simulink model "EJ_01_v18_02"  (R2018a)
settings: Solver=ode23t  StartTime=0.0  StopTime=5  FixedStep=0.01  MaxStep=0.05  RelTol=1e-3  EnableMultiTasking=on
PreLoadFcn:
  | mdl_puma560
values from neighbouring files (symbols this model uses):
  messi = SerialLink([links{:}], 'tool', Tool, 'name', 'messi')    [Ej_01.m]
  q0 = [0 -pi/2]    [Ej_01.m]
undefined symbols (not defined in the file or in its folder): jacob0, my_jacob, slcoulomb, vector_sweep
libraries: roblocks x5, dspmtrx3 x1
settings Model: ExtModeTrigMode=oneshot  ExtModeArmWhenConnect=off  Creator=pic  LastModifiedBy=sebas
settings SolverCC: ZeroCrossControl=DisableAll
settings DataIOCC: SaveFormat=Array  SignalLoggingSaveFormat=ModelDataLogs  ReturnWorkspaceOutputs=on  TimeSaveName=t  OutputSaveName=y  ReturnWorkspaceOutputsName=ctorque
settings OptimizationCC: BlockReduction=off  BooleanDataType=off  ExpressionDepthLimit=2147483647  InitFltsAndDblsToZero=on  LifeSpan=inf
settings DebuggingCC: SaveWithParameterizedLinksMsg=none  UnderspecifiedInitializationDetection=Classic  MergeDetectMultiDrivingBlocksExec=none  SignalResolutionControl=TryResolveAllWithWarning  MultiTaskDSMMsg=warning  MultiTaskCondExecSysMsg=none  FcnCallInpInsideContextMsg=warning  AllowSymbolicDim=off  StateNameClashWarn=warning  SFUnexpectedBacktrackingDiag=warning  SFNoUnconditionalDefaultTransitionDiag=warning  SFExecutionAtInitializationDiag=none
settings HardwareCC: ProdBitPerPointer=32  ProdBitPerSizeT=32  ProdBitPerPtrDiffT=32  ProdLargestAtomicFloat=None  ProdIntDivRoundTo=Undefined  ProdEndianess=Unspecified  ProdWordSize=32  ProdHWDeviceType=32-bit Generic  TargetUnknown=on
settings ModelReferenceCC: PropagateSignalLabelsOutOfModel=off
settings CodeAppCC: StateflowObjectComments=on
settings GRTTargetCC: TargetLangStandard=C89/C90 (ANSI)  ModelReferenceCompliant=off  CompOptLevelCompliant=off  GeneratePreprocessorConditionals=Disable all  CombineOutputUpdateFcns=off  MatFileLogging=off  GRTInterface=on
settings ConfigComp: CovMetricSettings=dw  CovHtmlReporting=on  CovSaveCumulativeToWorkspaceVar=on  CovSaveSingleToWorkspaceVar=on  CovExternalEMLEnable=off

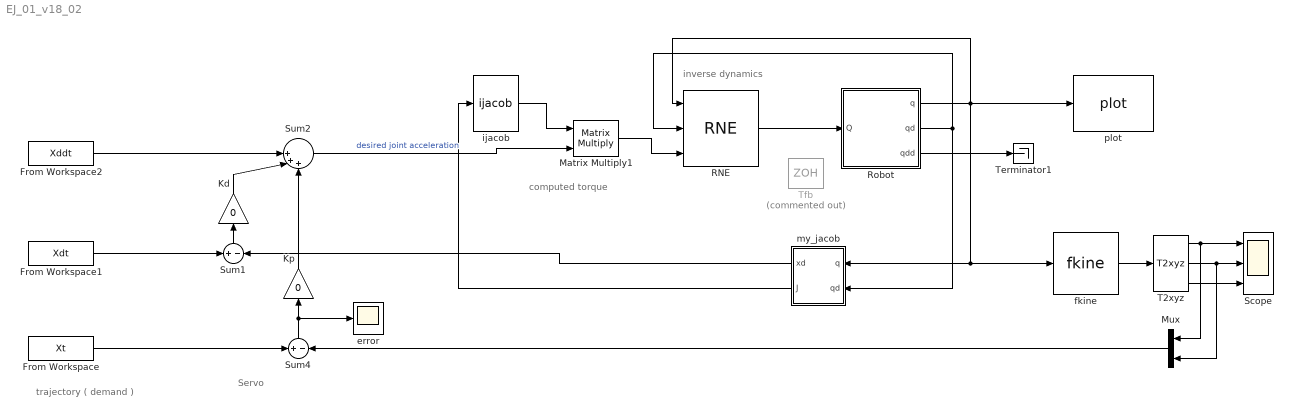
== system EJ_01_v18_02 ==
  note: inverse dynamics
  note: computed torque
  note: trajectory
      | ( demand )
  note: Servo
  From Workspace : FromWorkspace  VariableName=Xt
  From Workspace1 : FromWorkspace  VariableName=Xdt
  From Workspace2 : FromWorkspace  VariableName=Xddt
  Kd : Gain  Gain=0  SaturateOnIntegerOverflow=on  OutDataTypeStr=Inherit: Same as input  ParamDataTypeStr=Inherit: Same as input
  Kp : Gain  Gain=0  SaturateOnIntegerOverflow=on  OutDataTypeStr=Inherit: Same as input  ParamDataTypeStr=Inherit: Same as input
  Matrix Multiply1 : Product  Multiplication=Matrix(*)
  Mux : Mux  Inputs=2
  RNE : roblocks/Arm/RNE  robot=messi  grav=[0 0 9.81]
  Robot : Subsystem  AncestorBlock=roblocks/Arm/Robot  mask{robot=messi, q0=q0}
      mask prompts: robot "Robot object"; q0 "Initial state"
      mask help: Rigid-body dynamic model of robot.
      mask init:
      | if isa(robot, 'SerialLink')
      |     rname = robot.name;
      |     %fprintf('**robot name is %s\n', rname);
      | else
      |     rname = '';
      |     n = 0
      | end
      mask Help:
      | Simulates the forward (direct) rigid-body dynamics of the robot described
      | by the given robot object.  For given applied joint torque/force it computes
      | the instaneous joint coordinates, velocities and acclerations.
      | 
      | 
      | <b>Parameters::</b>
      | 
      | robot (SerialLink) a dynamic model of an N-link serial link manipulator
      | q0 (1xN)  Initial joint coordinates
      | 
      | <b>Inputs::</b>
      | 
      | Q (1xN) the generalized joint force (torque or force) required to achieve
      | the motion state (q, qd, qdd).
      | 
      | <b>Outputs::</b>
      | 
      | q (1xN) joint coordinates
      | qd (1xN) joint coordinate velocity
      | qdd (1xN) joint coordinate acceleration
      | 
      | 
      | <b>Notes::</b>
      | 
      | - Required to simulate robot rigid body motion.
      | - Implemented using the recursive Newton-Euler scheme (RNE).
      | - A wrapper for the Toolbox method accel() which in turn depends on the
      |   method rne().
      mask Display:
      | port_label('input', 1, 'Q')
      | port_label('output', 1, 'q')
      | port_label('output', 2, 'qd')
      | port_label('output', 3, 'qdd')
      | text(0.1, 0.9,  rname, 'horizontalAlignment', 'left')
  Scope : Scope  NumInputPorts=3
  Sum1 : Sum  Inputs=+|-  SaturateOnIntegerOverflow=on  InputSameDT=on  OutDataTypeStr=Inherit: Same as first input
  Sum2 : Sum  Inputs=||+++  SaturateOnIntegerOverflow=on  InputSameDT=on  OutDataTypeStr=Inherit: Same as first input
  Sum4 : Sum  Inputs=+|-  SaturateOnIntegerOverflow=on  InputSameDT=on  OutDataTypeStr=Inherit: Same as first input
  T2xyz : roblocks/Toolbox/T2xyz
  Terminator1 : Terminator
  Tfb : ZeroOrderHold  Commented=on  SampleTime=0.005
  error : Scope
  fkine : roblocks/Arm/fkine  robot=messi
  ijacob : roblocks/Arm/ijacob
  "my_jacob " : Subsystem  AncestorBlock=vector_sweep/my_jacob  mask{robot=messi}
      mask prompts: robot "Robot object"
      mask help: Robot Jacobian in world coordinates
      mask init:
      | n=robot.n;
      mask Help:
      | Jacobian matrix relating joint coordinate rates to end-effector spatial
      | velocity expressed in the world frame.
      | 
      | <b>Parameters::</b>
      | 
      | Robot (SerialLink class)  The N-axis robot object for which the Jacobian is
      |                           computed.
      | 
      | <b>Inputs::</b>
      | 
      | q (1xN) joint coordinates
      | 
      | <b>Outputs::</b>
      | 
      | J (6xN) the Jacobian matrix
      | 
      | <b>Notes::</b>
      | 
      | - A wrapper for the Toolbox method jacob0().
      mask Display:
      | text(0.4, 0.7, '\bf\fontsize{16}J', 'texmode', 'on', 'verticalAlignment', 'top', 'horizontalAlignment', 'left')
      | text(0.45, 0.65, '\fontsize{10}0', 'texmode', 'on','verticalAlignment', 'bottom', 'horizontalAlignment', 'right')
      | if ~isempty(robot)
      |     text(0.5, 0.2, robot.name,  'horizontalAlignment', 'center')
      | end
      | port_label('input', 1, 'q')
      | port_label('input', 2, 'qd')
      | port_label('output', 1, 'xd')
  plot : roblocks/Arm/plot  robot=messi  fps=10  holdplot=on
  wires:
  Robot/3(qdd) -> Terminator1/1
  fkine/1 -> T2xyz/1
  T2xyz/3 -> Scope/3
  T2xyz/2 -> Mux/2, Scope/2
  T2xyz/1 -> Mux/1, Scope/1
  Sum1/1 -> Kd/1
  Sum4/1 -> Kp/1, error/1
  From Workspace/1 -> Sum4/1
  From Workspace1/1 -> Sum1/1
  Kp/1 -> Sum2/3
  Kd/1 -> Sum2/2
  From Workspace2/1 -> Sum2/1
  RNE/1 -> Robot/1(Q)
  Mux/1 -> Sum4/2
  "my_jacob "/1(xd) -> Sum1/2
  ijacob/1 -> Matrix Multiply1/1
  Sum2/1 -> Matrix Multiply1/2  "desired joint acceleration"
  Matrix Multiply1/1 -> RNE/3
  Robot/1(q) -> plot/1, fkine/1, "my_jacob "/1(q), RNE/1
  Robot/2(qd) -> "my_jacob "/2(qd), RNE/2
  "my_jacob "/2(J) -> ijacob/1

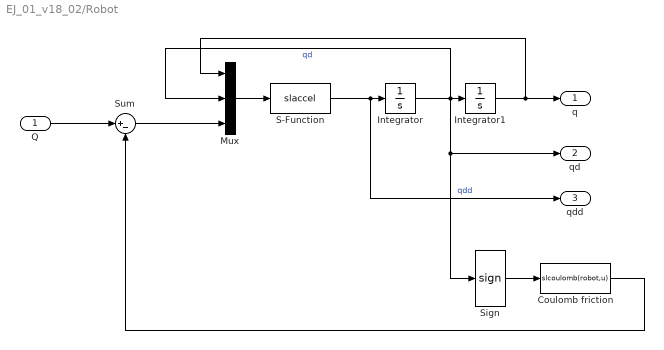
== system EJ_01_v18_02/Robot ==
  Q : Inport
  Coulomb friction : MATLABFcn  MATLABFcn=slcoulomb(robot,u)  OutputDimensions=[robot.n 1]  Output1D=off
  Integrator : Integrator
  Integrator1 : Integrator  InitialCondition=q0
  Mux : Mux  Inputs=3
  S-Function : S-Function  FunctionName=slaccel  Parameters=robot  SFunctionDeploymentMode=off  EnableBusSupport=off
  Sign : Signum
  Sum : Sum  Inputs=|+-
  q : Outport
  qd : Outport  Port=2
  qdd : Outport  Port=3
  wires:
  S-Function/1 -> qdd/1, Integrator/1  "qdd"
  Mux/1 -> S-Function/1
  Integrator/1 -> Sign/1, qd/1, Integrator1/1, Mux/2  "qd"
  Integrator1/1 -> q/1, Mux/1
  Q/1 -> Sum/1
  Sum/1 -> Mux/3
  Coulomb friction/1 -> Sum/2
  Sign/1 -> Coulomb friction/1

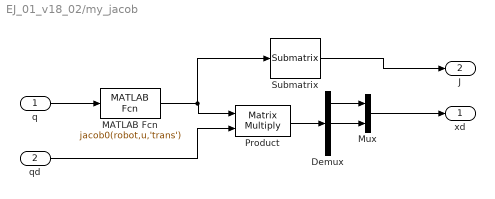
== system EJ_01_v18_02/my_jacob  ==
  q : Inport
  qd : Inport  Port=2
  Demux : Demux  Outputs=3
  MATLAB Fcn : MATLABFcn  MATLABFcn=jacob0(robot,u,'trans')  Output1D=off
  Mux : Mux  Inputs=2
  Product : Product  Multiplication=Matrix(*)
  Submatrix : dspmtrx3/Submatrix  RowSpan=Range of rows  RowStartMode=First  RowStartIndex=1  RowEndMode=Index  RowEndIndex=2  ColSpan=Range of columns  ColStartMode=First  ColStartIndex=1  ColEndMode=Index  ColEndIndex=2
  xd : Outport
  J : Outport  Port=2
  wires:
  Product/1 -> Demux/1
  qd/1 -> Product/2
  q/1 -> MATLAB Fcn/1
  MATLAB Fcn/1 -> Submatrix/1, Product/1
  Demux/2 -> Mux/2
  Demux/1 -> Mux/1
  Mux/1 -> xd/1
  Submatrix/1 -> J/1
